simulink model "DiskreterPID_Pan"  (R2022a)
settings: Solver=VariableStepAuto  StartTime=0.0  StopTime=10.0  RelTol=1e-3
values from neighbouring files (symbols this model uses):
  DT = 0.2    [AuslegungZieglerNichols.m]
  ki = kp/(3.33*T_t)    (= 2.09315698677)    [AuslegungZieglerNichols.m]
  kp = (0.9/K)*(T/T_t)    (= 0.697021276596)    [AuslegungZieglerNichols.m]
  T = 0.091    [AuslegungZieglerNichols.m]
undefined symbols (not defined in the file or in its folder): kd
libraries: slpidlib x1, cstblocks x1
settings Model: Creator=Uni  LastModifiedBy=Uni

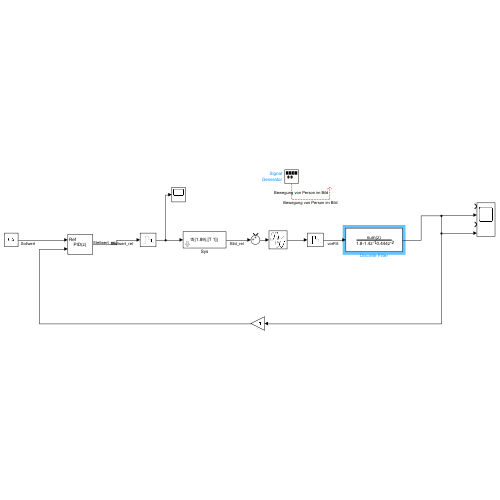
[thumbnail: Simulink's stored preview of the top-level diagram]
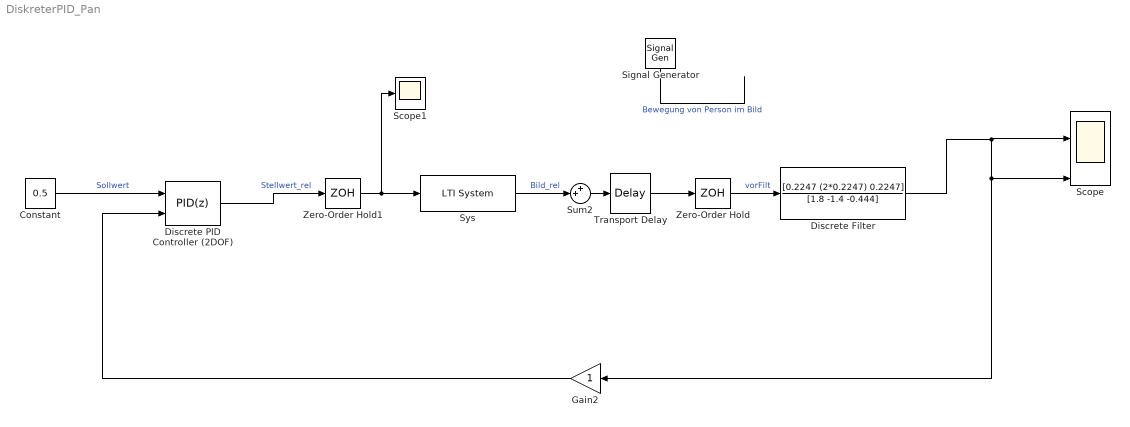
== system DiskreterPID_Pan ==
  Constant : Constant  Value=0.5
  Discrete Filter : DiscreteFilter  Numerator=[0.2247 (2*0.2247) 0.2247]  Denominator=[1.8 -1.4 -0.444]  SampleTime=DT
  Discrete PID Controller (2DOF) : slpidlib/PID Controller (2DOF)  Controller=PID  Form=Parallel  TimeDomain=Discrete-time  UseExternalTs=off  SampleTime=-1  IntegratorMethod=Forward Euler  FilterMethod=Forward Euler  ControllerParametersSource=internal  P=kp  I=ki  UseKiTs=off  D=kd  N=100  UseFilter=off  b=1  c=1  TunerSelectOption=Transfer Function Based (PID Tuner App)  InitialConditionSource=internal  InitialConditionForIntegrator=0  InitialConditionForFilter=0  DifferentiatorICPrevScaledInput=0  ExternalReset=none  TrackingMode=off  Kt=1  LimitOutput=off  SatLimitsSource=internal  UpperSaturationLimit=inf  LowerSaturationLimit=-inf  LinearizeAsGain=off  AntiWindupMode=none  Kb=1  POutMin=[]  POutMax=[]  IOutMin=[]  IOutMax=[]  DOutMin=[]  DOutMax=[]  NOutMin=[]  NOutMax=[]  bOutMin=[]  bOutMax=[]  cOutMin=[]  cOutMax=[]  SumOutMin=[]  SumOutMax=[]  SaturationOutMin=[]  SaturationOutMax=[]  PParamMin=[]  PParamMax=[]  IParamMin=[]  IParamMax=[]  DParamMin=[]  DParamMax=[]  NParamMin=[]  NParamMax=[]  bParamMin=[]  bParamMax=[]  cParamMin=[]  cParamMax=[]  KbParamMin=[]  KbParamMax=[]  KtParamMin=[]  KtParamMax=[]  KbOutMin=[]  KbOutMax=[]  KtOutMin=[]  KtOutMax=[]  IntegratorOutMin=[]  IntegratorOutMax=[]  FilterOutMin=[]  FilterOutMax=[]  SumI1OutMin=[]  SumI1OutMax=[]  SumI2OutMin=[]  SumI2OutMax=[]  SumI3OutMin=[]  SumI3OutMax=[]  SumI4OutMin=[]  SumI4OutMax=[]  SumDOutMin=[]  SumDOutMax=[]  Sum1OutMin=[]  Sum1OutMax=[]  Sum2OutMin=[]  Sum2OutMax=[]  Sum3OutMin=[]  Sum3OutMax=[]  DifferentiatorOutMin=[]  DifferentiatorOutMax=[]  FilterDiffOutCoefMin=[]  FilterDiffOutCoefMax=[]  ReciprocalOutMin=[]  ReciprocalOutMax=[]  SumDenOutMin=[]  SumDenOutMax=[]  SumNumOutMin=[]  SumNumOutMax=[]  DivideOutMin=[]  DivideOutMax=[]  UdiffTsProdOutMin=[]  UdiffTsProdOutMax=[]  NTsProdOutMin=[]  NTsProdOutMax=[]  UintegralTsProdOutMin=[]  UintegralTsProdOutMax=[]  UngainTsProdOutMin=[]  UngainTsProdOutMax=[]  IntegratorContinuousStateAttributes=''  IntegratorStateMustResolveToSignalObject=off  IntegratorRTWStateStorageClass=Auto  FilterContinuousStateAttributes=''  FilterStateMustResolveToSignalObject=off  FilterRTWStateStorageClass=Auto  ParallelPVariant=InternalParameters  IdealPVariant=Disabled  IVariant=InternalParameters  DVariant=InternalParameters  bVariant=InternalParameters  cVariant=InternalParameters  IntegratorVariant=Discrete  SatVariant=Disabled  AWVariant=Passthrough  PCopyVariant=Disabled  TRVariant=Disabled  FdbkBlocksVariant=Forward  IdealPFdbkVariant=Disabled  SatFdbkVariant=Disabled  DerivativeFilterVariant=Differentiator  NVariant=Passthrough  NCopyVariant=Disabled_SignalSpec  FilterICVariant=InternalICsDifferentiator  IntegratorICVariant=InternalICs  ExternalResetVariant=Disabled  TRSumVariant=Passthrough  SumFdbkVariant=Disabled  SumVariant=Sum_PID  TsampFilterVariant=InternalTs  TsampNgainVariant=Passthrough  TsampIntegralVariant=Passthrough  ExternalSaturationOutDataTypeStr=Inherit: Same as second input
      settings: SourceProductBaseCode=SL
  Gain2 : Gain
  Scope : Scope  NumInputPorts=4
  Scope1 : Scope
  Signal Generator : SignalGenerator  Amplitude=0.2  Units=rad/sec
  Sum2 : Sum  Inputs=++|
  Sys : cstblocks/LTI System  sys=tf((1.89),[T 1])  IC=[]
  Transport Delay : TransportDelay  DelayTime=DT
  Zero-Order Hold : ZeroOrderHold  SampleTime=DT
  Zero-Order Hold1 : ZeroOrderHold  SampleTime=DT
  wires:
  Zero-Order Hold1/1 -> Scope1/1, Sys/1
  Transport Delay/1 -> Zero-Order Hold/1
  Sys/1 -> Sum2/2  "Bild_rel"
  Signal Generator/1 -> ?  "Bewegung von Person im Bild"
  Sum2/1 -> Transport Delay/1
  Discrete PID Controller (2DOF)/1 -> Zero-Order Hold1/1  "Stellwert_rel"
  Constant/1 -> Discrete PID Controller (2DOF)/1  "Sollwert"
  Zero-Order Hold/1 -> Discrete Filter/1  "vorFilt"
  Gain2/1 -> Discrete PID Controller (2DOF)/2
  Discrete Filter/1 -> Gain2/1, Scope/4, Scope/2
